simulink model "p4_2_1"  (R2016a)
settings: Solver=VariableStepAuto  StartTime=0.0  StopTime=10.0  RelTol=1e-3
settings Model: Creator=maximilian  LastModifiedBy=maximilian

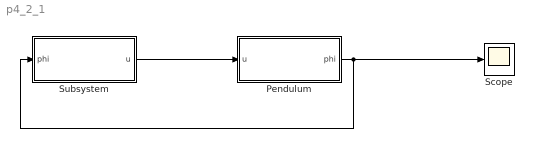
== system p4_2_1 ==
  Pendulum : Subsystem
  Scope : Scope
  Subsystem : Subsystem
  wires:
  Subsystem/1(u) -> Pendulum/1("u ")
  Pendulum/1(phi) -> Scope/1, Subsystem/1(phi)

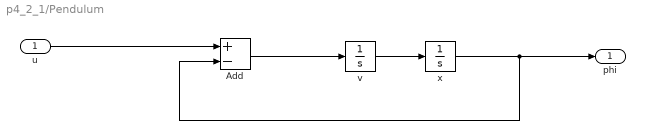
== system p4_2_1/Pendulum ==
  "u " : Inport
  Add : Sum  Inputs=+-
  v : Integrator
  x : Integrator  InitialCondition=2
  phi : Outport
  wires:
  "u "/1 -> Add/1
  Add/1 -> v/1
  v/1 -> x/1
  x/1 -> Add/2, phi/1

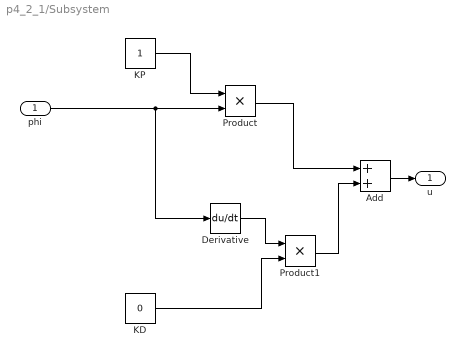
== system p4_2_1/Subsystem ==
  phi : Inport
  Add : Sum
  Derivative : Derivative
  KD : Constant  Value=0
  KP : Constant
  Product : Product
  Product1 : Product
  u : Outport
  wires:
  KP/1 -> Product/1
  Product/1 -> Add/1
  Add/1 -> u/1
  KD/1 -> Product1/2
  Derivative/1 -> Product1/1
  Product1/1 -> Add/2
  phi/1 -> Derivative/1, Product/2
